simulink model "rtwdemo_f14"  (Simulink 6.0)
settings: Solver=ode3  StartTime=0.0  StopTime=60  RelTol=1e-4  AbsTol=1e-6
PreLoadFcn:
  | f14dat
values from neighbouring files (symbols this model uses):
  g = 32.2    [rtwdemo_eml_aero_radar_data.m]
  Ki = Simulink.Parameter    [rtwdemo_capi_data.m]
undefined symbols (not defined in the file or in its folder): a, b, Ka, Kf, Kq, Md, Mq, Mw, Swg, Ta, Tal, Ts, Uo, Vto, W1, W2, Zd, Zw
libraries: rtwdemowidgets x1, simulink x1
settings Model: Creator=The MathWorks Inc.  LastModifiedBy=batserve  ExtModeTrigMode=oneshot  ExtModeArmWhenConnect=off  ExtModeAutoUpdateStatusClock=off
settings SolverCC: AutoInsertRateTranBlk=on
settings DataIOCC: ExternalInput=[]  InitialState=[]  LimitDataPoints=off  SaveOutput=off  SaveTime=off  SignalLoggingName=logsOut
settings OptimizationCC: InlineParams=on  EnforceIntegerDowncast=off  StateBitsets=on  DataBitsets=on  UseTempVars=on
settings DebuggingCC: CheckExecutionContextPreStartOutputMsg=on  CheckExecutionContextRuntimeOutputMsg=on  SolverPrmCheckMsg=none  IntegerOverflowMsg=none
settings ModelReferenceCC: UpdateModelReferenceTargets=IfOutOfDate
settings RTWCC: TLCOptions=-p0 -aWarnNonSaturatedBlocks=0  GenerateReport=on  RTWVerbose=off  ProcessScript=grt_make_rtw_hook  LaunchReport=on
settings CodeAppCC: ForceParamTrailComments=on
settings GRTTargetCC: MatFileLogging=off

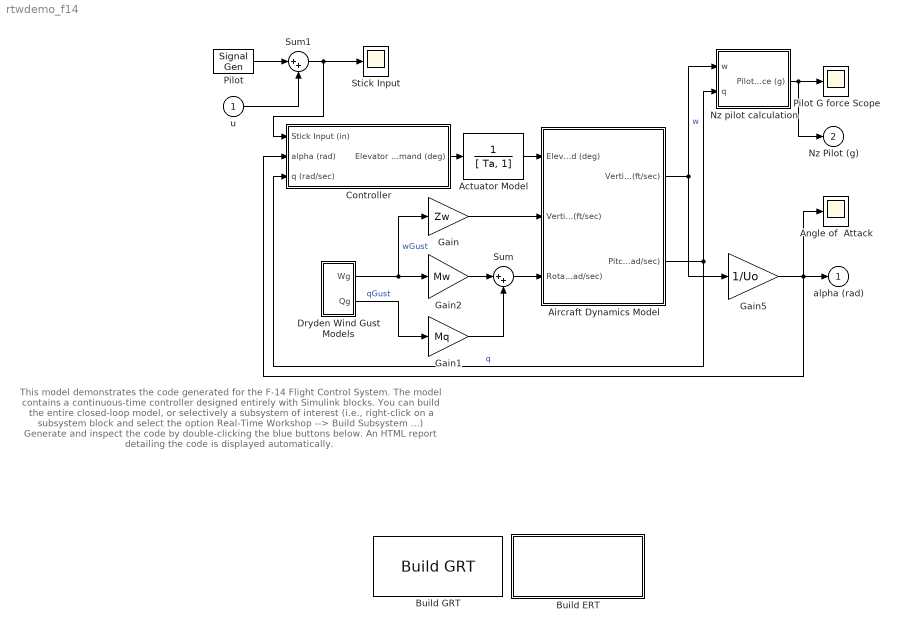
== system rtwdemo_f14 ==
  note: This model demonstrates the code generated for the F-14 Flight Control System.  The model contains
      | a continuous-time controller designed entirely with Simulink blocks.  You can build the entire
      | closed-loop model, or selectively a subsystem of interest (i.e., right-click on a subsystem block and
      | select the option Real-Time Workshop --> Build Subsystem ...)
      |
      | Generate and inspect the code by double-clicking the blue buttons below.  An HTML report detailing
      | the code is displayed automatically.
  u : Inport  Port=1  LatchInput=off
  Actuator Model : TransferFcn  Denominator=[ Ta, 1]
  Aircraft Dynamics Model : Subsystem  PropExecContextAcrossSSBoundary=on
  Angle of  Attack : Scope
      settings: TickLabels=on  TimeRange=60  YMin=-1.25  YMax=1.25  DataFormat=Array
  Build ERT : Subsystem  AncestorBlock=rtwdemowidgets/Build ERT  PropExecContextAcrossSSBoundary=on  mask{attrib_overrides={}}
      mask prompts: attrib_overrides "List of attributes to preserve (cell of strings):"
      mask help: Enter the attributes of the configuration set that you want preserved. Otherwise, the default configuration script will override your current settings.
      settings: OpenFcn=|
      | model=bdroot;
      | overrides=get_param(gcb,'attrib_overrides');
      | try
      |   rtwconfiguredemo(model,'noop',false,overrides);
      |   cs = getActiveConfigSet(model);
      |   set_param(cs,'SupportNonFinite','on');
      |   rtwbuilddemomodel(model);
      | catch
      |   error(lasterr);
      | end
      mask Display:
      | disp(['Generate Code Using\n',...
      | 	  'Real-Time Workshop\n',...
      | 	  'Embedded Coder\n'...
      | 	  '(double-click)'])
  Build GRT : rtwdemowidgets/Build GRT  attrib_overrides={}
  Controller : Subsystem  PropExecContextAcrossSSBoundary=on
  Dryden Wind Gust Models : Subsystem  PropExecContextAcrossSSBoundary=on
  Gain : Gain  Gain=Zw  SaturateOnIntegerOverflow=on
  Gain1 : Gain  Gain=Mq  SaturateOnIntegerOverflow=on
  Gain2 : Gain  Gain=Mw  SaturateOnIntegerOverflow=on
  Gain5 : Gain  Gain=1/Uo  SaturateOnIntegerOverflow=on
  Nz pilot calculation : Subsystem  PropExecContextAcrossSSBoundary=on
  Pilot : SignalGenerator  WaveForm=square  Frequency=0.500000  Units=rad/sec
  Pilot G force Scope : Scope
      settings: TickLabels=on  TimeRange=60  YMin=-15  YMax=15  DataFormat=Array
  Stick Input : Scope
      settings: TickLabels=on  TimeRange=60  YMin=-1.5  YMax=1.5  DataFormat=Array
  Sum : Sum  Inputs=|++  SaturateOnIntegerOverflow=on  InputSameDT=on
  Sum1 : Sum  Inputs=|++  SaturateOnIntegerOverflow=on  InputSameDT=on
  alpha (rad) : Outport  InitialOutput=0
  Nz Pilot (g) : Outport  Port=2  InitialOutput=0
  wires:
  Gain5/1 -> alpha (rad)/1, Angle of  Attack/1, Controller/2(alpha (rad))
  Aircraft Dynamics Model/1(Vertical Velocity w (ft/sec)) -> Gain5/1, Nz pilot calculation/1(w)  "w"
  Nz pilot calculation/1(Pilot g force (g)) -> Pilot G force Scope/1, Nz Pilot (g)/1
  Gain2/1 -> Sum/1
  Gain/1 -> Aircraft Dynamics Model/2(Vertical Gust wGust (ft/sec))
  Pilot/1 -> Sum1/1
  u/1 -> Sum1/2
  Dryden Wind Gust Models/2(Qg) -> Gain1/1  "qGust"
  Dryden Wind Gust Models/1(Wg) -> Gain2/1, Gain/1  "wGust"
  Sum/1 -> Aircraft Dynamics Model/3(Rotary Gust qGust (rad/sec))
  Gain1/1 -> Sum/2
  Aircraft Dynamics Model/2(Pitch Rate q (rad/sec)) -> Nz pilot calculation/2(q), Controller/3(q (rad/sec))  "q"
  Actuator Model/1 -> Aircraft Dynamics Model/1(Elevator Deflection d (deg))
  Controller/1(Elevator Command (deg)) -> Actuator Model/1
  Sum1/1 -> Stick Input/1, Controller/1(Stick Input (in))

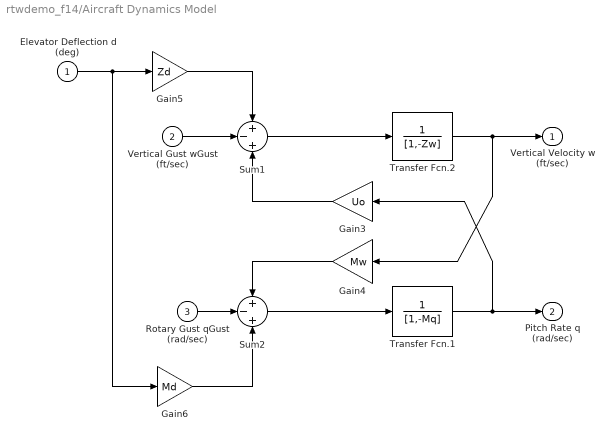
== system rtwdemo_f14/Aircraft Dynamics Model ==
  Elevator Deflection d (deg) : Inport  Port=1  LatchInput=off
  Vertical Gust wGust (ft/sec) : Inport  Port=2  LatchInput=off
  Rotary Gust qGust (rad/sec) : Inport  Port=3  LatchInput=off
  Gain3 : Gain  Orientation=left  Gain=Uo  SaturateOnIntegerOverflow=on
  Gain4 : Gain  Orientation=left  Gain=Mw  SaturateOnIntegerOverflow=on
  Gain5 : Gain  Gain=Zd  SaturateOnIntegerOverflow=on
  Gain6 : Gain  Gain=Md  SaturateOnIntegerOverflow=on
  Sum1 : Sum  Inputs=+-+  SaturateOnIntegerOverflow=on  InputSameDT=on
  Sum2 : Sum  Inputs=+-+  SaturateOnIntegerOverflow=on  InputSameDT=on
  Transfer Fcn.1 : TransferFcn  Denominator=[1,-Mq]
  Transfer Fcn.2 : TransferFcn  Denominator=[1,-Zw]
  Vertical Velocity w (ft/sec) : Outport  InitialOutput=0
  Pitch Rate q (rad/sec) : Outport  Port=2  InitialOutput=0
  wires:
  Transfer Fcn.2/1 -> Vertical Velocity w (ft/sec)/1, Gain4/1
  Transfer Fcn.1/1 -> Pitch Rate q (rad/sec)/1, Gain3/1
  Gain6/1 -> Sum2/3
  Gain5/1 -> Sum1/1
  Gain3/1 -> Sum1/3
  Rotary Gust qGust (rad/sec)/1 -> Sum2/2
  Sum2/1 -> Transfer Fcn.1/1
  Sum1/1 -> Transfer Fcn.2/1
  Gain4/1 -> Sum2/1
  Vertical Gust wGust (ft/sec)/1 -> Sum1/2
  Elevator Deflection d (deg)/1 -> Gain5/1, Gain6/1

== system rtwdemo_f14/Build ERT ==

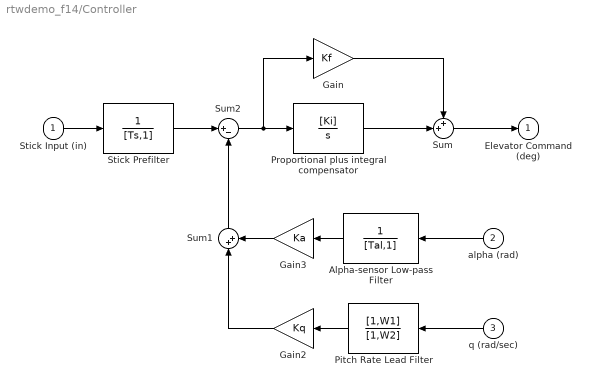
== system rtwdemo_f14/Controller ==
  Stick Input (in) : Inport  Port=1  LatchInput=off
  alpha (rad) : Inport  Orientation=left  Port=2  LatchInput=off
  q (rad/sec) : Inport  Orientation=left  Port=3  LatchInput=off
  Alpha-sensor Low-pass Filter : TransferFcn  Orientation=left  Denominator=[Tal,1]
  Gain : Gain  Gain=Kf  SaturateOnIntegerOverflow=on
  Gain2 : Gain  Orientation=left  Gain=Kq  SaturateOnIntegerOverflow=on
  Gain3 : Gain  Orientation=left  Gain=Ka  SaturateOnIntegerOverflow=on
  Pitch Rate Lead Filter : TransferFcn  Orientation=left  Numerator=[1,W1]  Denominator=[1,W2]
  Proportional plus integral compensator : TransferFcn  Numerator=[Ki]  Denominator=[1,0]
  Stick Prefilter : TransferFcn  Denominator=[Ts,1]
  Sum : Sum  Inputs=++|  SaturateOnIntegerOverflow=on  InputSameDT=on
  Sum1 : Sum  Orientation=up  Inputs=|++  SaturateOnIntegerOverflow=on  InputSameDT=on
  Sum2 : Sum  Inputs=|+-  SaturateOnIntegerOverflow=on  InputSameDT=on
  Elevator Command (deg) : Outport  InitialOutput=0
  wires:
  Sum2/1 -> Proportional plus integral compensator/1, Gain/1
  Gain/1 -> Sum/1
  Proportional plus integral compensator/1 -> Sum/2
  Stick Prefilter/1 -> Sum2/1
  Sum/1 -> Elevator Command (deg)/1
  Gain2/1 -> Sum1/1
  Gain3/1 -> Sum1/2
  Sum1/1 -> Sum2/2
  Pitch Rate Lead Filter/1 -> Gain2/1
  q (rad/sec)/1 -> Pitch Rate Lead Filter/1
  Alpha-sensor Low-pass Filter/1 -> Gain3/1
  alpha (rad)/1 -> Alpha-sensor Low-pass Filter/1
  Stick Input (in)/1 -> Stick Prefilter/1

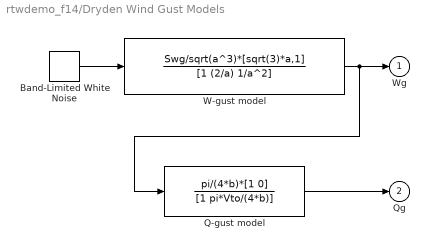
== system rtwdemo_f14/Dryden Wind Gust Models ==
  Band-Limited White Noise : simulink/Sources/Band-Limited White Noise  Cov=1  Ts=0.1  seed=[23341]
  Q-gust model : TransferFcn  Numerator=pi/(4*b)*[1 0]  Denominator=[1 pi*Vto/(4*b)]
  W-gust model : TransferFcn  Numerator=Swg/sqrt(a^3)*[sqrt(3)*a,1]  Denominator=[1 (2/a) 1/a^2]
  Wg : Outport  InitialOutput=0
  Qg : Outport  Port=2  InitialOutput=0
  wires:
  Band-Limited White Noise/1 -> W-gust model/1
  Q-gust model/1 -> Qg/1
  W-gust model/1 -> Wg/1, Q-gust model/1

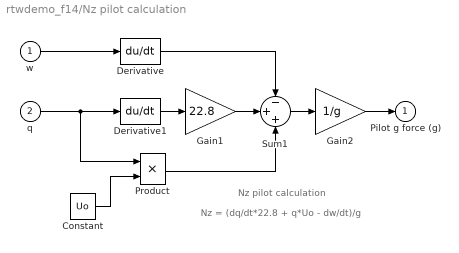
== system rtwdemo_f14/Nz pilot calculation ==
  note: Nz pilot calculation
  note: Nz = (dq/dt*22.8 + q*Uo - dw/dt)/g
  w : Inport  Port=1  LatchInput=off
  q : Inport  Port=2  LatchInput=off
  Constant : Constant  Value=Uo
  Derivative : Derivative
  Derivative1 : Derivative
  Gain1 : Gain  Gain=22.8  SaturateOnIntegerOverflow=on
  Gain2 : Gain  Gain=1/g  SaturateOnIntegerOverflow=on
  Product : Product  SaturateOnIntegerOverflow=on  RndMeth=Zero  InputSameDT=on
  Sum1 : Sum  Inputs=-++  SaturateOnIntegerOverflow=on  InputSameDT=on
  Pilot g force (g) : Outport  InitialOutput=0
  wires:
  q/1 -> Product/1, Derivative1/1
  Constant/1 -> Product/2
  Gain2/1 -> Pilot g force (g)/1
  Sum1/1 -> Gain2/1
  Derivative1/1 -> Gain1/1
  Gain1/1 -> Sum1/2
  Product/1 -> Sum1/3
  Derivative/1 -> Sum1/1
  w/1 -> Derivative/1
